simulink model "GPC_GUI"  (R2015b)
settings: Solver=FixedStepAuto  StartTime=0.0  StopTime=100  FixedStep=0.2  RelTol=1e-3
settings Model: Creator=E:\GreenSoftware\TDZ\User\  LastModifiedBy=TroyLab

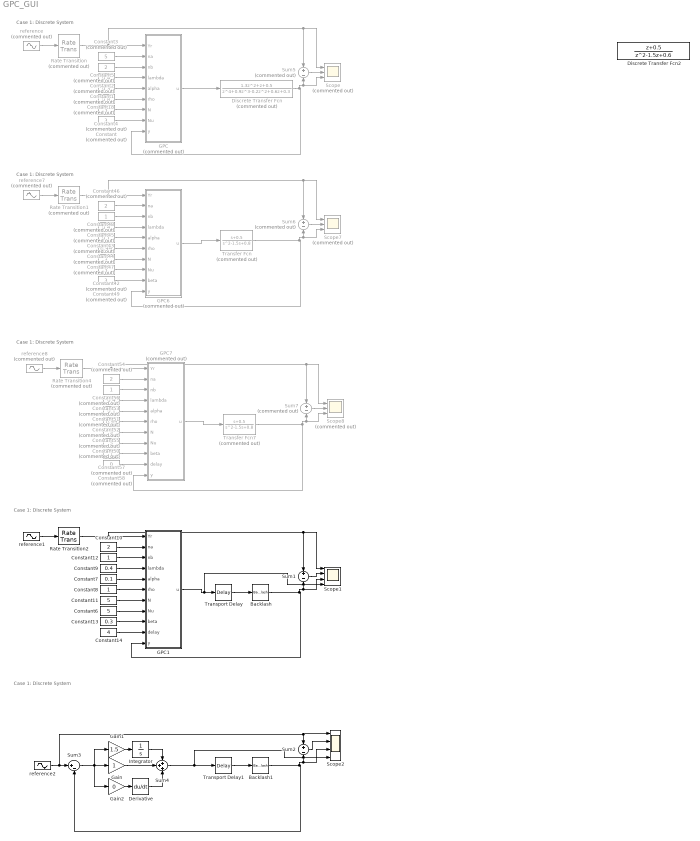
== system GPC_GUI ==
  note: Case 1: Discrete System
  note: Case 1: Discrete System
  note: Case 1: Discrete System
  note: Case 1: Discrete System
  note: Case 1: Discrete System
  Backlash : Backlash  BacklashWidth=1.5
  Backlash1 : Backlash
  Constant{,4,42,47,49} (5 alike) : Constant  Commented=on  Value=3
  Constant1 : Constant  Commented=on  Value=0.3
  Constant10 : Constant  Value=2
  Constant11 : Constant  Value=5
  Constant12 : Constant
  Constant13 : Constant  Value=0.3
  Constant14 : Constant  Value=4
  Constant18 : Constant  Commented=on  Value=0.8
  Constant2 : Constant  Commented=on  Value=0.4
  Constant3 : Constant  Commented=on  Value=5
  Constant43 : Constant  Commented=on  Value=0.1
  Constant44 : Constant  Commented=on  Value=0.99
  Constant45 : Constant  Commented=on  Value=0.4
  Constant46 : Constant  Commented=on  Value=2
  Constant48 : Constant  Commented=on
  Constant5 : Constant  Commented=on  Value=2
  Constant50 : Constant  Commented=on  Value=5
  Constant51 : Constant  Commented=on  Value=0.1
  Constant52 : Constant  Commented=on  Value=0.99
  Constant53 : Constant  Commented=on  Value=0.4
  Constant54 : Constant  Commented=on  Value=2
  Constant55 : Constant  Commented=on  Value=5
  Constant56 : Constant  Commented=on
  Constant57 : Constant  Commented=on
  Constant58 : Constant  Commented=on  Value=0
  Constant6 : Constant  Value=5
  Constant7 : Constant  Value=0.1
  Constant8 : Constant
  Constant9 : Constant  Value=0.4
  Derivative : Derivative
  Discrete Transfer Fcn : DiscreteTransferFcn  Commented=on  Numerator=[1.3, 1, 0.5]  Denominator=[1, 0.9, -0.2, 0.6, 0.3]
  Discrete Transfer Fcn2 : DiscreteTransferFcn  Numerator=[1, 0.5]  Denominator=[1, -1.5, 0.6]
  GPC : MATLAB Function  Commented=on  TreatAsAtomicUnit=on
  GPC1 : MATLAB Function  TreatAsAtomicUnit=on
  GPC6 : MATLAB Function  Commented=on  TreatAsAtomicUnit=on
  GPC7 : MATLAB Function  Commented=on  TreatAsAtomicUnit=on
  Gain : Gain
  Gain1 : Gain  Gain=1.5
  Gain2 : Gain  Gain=0
  Integrator : Integrator
  Rate Transition : RateTransition  Commented=on
  Rate Transition1 : RateTransition  Commented=on
  Rate Transition2 : RateTransition
  Rate Transition4 : RateTransition  Commented=on
  Scope : Scope  Commented=on  NumInputPorts=3
  Scope1 : Scope  NumInputPorts=4
  Scope2 : Scope  NumInputPorts=4
  Scope7 : Scope  Commented=on  NumInputPorts=3
  Scope8 : Scope  Commented=on  NumInputPorts=3
  Sum1 : Sum  Inputs=+|-
  Sum2 : Sum  Inputs=+|-
  Sum3 : Sum  Inputs=|+-
  Sum4 : Sum  Inputs=+++
  Sum5 : Sum  Commented=on  Inputs=+|-
  Sum6 : Sum  Commented=on  Inputs=+|-
  Sum7 : Sum  Commented=on  Inputs=+|-
  Transfer Fcn : TransferFcn  Commented=on  Numerator=[1, 0.5]  Denominator=[1, -1.5, 0.8]
  Transfer Fcn7 : TransferFcn  Commented=on  Numerator=[1, 0.5]  Denominator=[1, -1.5, 0.8]
  Transport Delay : TransportDelay  DelayTime=0.6
  Transport Delay1 : TransportDelay  DelayTime=0.6
  reference : Sin  Commented=on  Frequency=0.2  Phase=pi/4  SampleTime=0
  reference1 : Sin  Amplitude=10  Frequency=0.5  Phase=pi/4  SampleTime=0
  reference2 : Sin  Amplitude=10  Frequency=0.5  Phase=pi/4  SampleTime=0
  reference7 : Sin  Commented=on  Amplitude=10  Frequency=0.5  Phase=pi/4  SampleTime=0
  reference8 : Sin  Commented=on  Amplitude=10  Frequency=0.5  Phase=pi/4  SampleTime=0
  wires:
  reference/1 -> Rate Transition/1
  Constant/1 -> GPC/8(Nu)
  Constant1/1 -> GPC/5(alpha)
  Constant2/1 -> GPC/4(lambda)
  Constant3/1 -> GPC/2(na)
  Constant4/1 -> GPC/7(N)
  Constant5/1 -> GPC/3(nb)
  Discrete Transfer Fcn/1 -> Sum5/2, Scope/3, GPC/9(y)
  Rate Transition/1 -> Sum5/1, Scope/1, GPC/1(Yr)
  GPC/1(u) -> Discrete Transfer Fcn/1
  Transport Delay/1 -> Backlash/1
  Constant18/1 -> GPC/6(rho)
  Sum5/1 -> Scope/2
  reference7/1 -> Rate Transition1/1
  Constant42/1 -> GPC6/8(Nu)
  Constant43/1 -> GPC6/5(alpha)
  Constant45/1 -> GPC6/4(lambda)
  Constant46/1 -> GPC6/2(na)
  Constant47/1 -> GPC6/7(N)
  Constant48/1 -> GPC6/3(nb)
  Transfer Fcn/1 -> GPC6/10(y), Scope7/3, Sum6/2
  Rate Transition1/1 -> GPC6/1(Yr), Scope7/1, Sum6/1
  GPC6/1(u) -> Transfer Fcn/1
  Constant44/1 -> GPC6/6(rho)
  Sum6/1 -> Scope7/2
  Constant49/1 -> GPC6/9(beta)
  reference8/1 -> Rate Transition4/1
  Constant50/1 -> GPC7/8(Nu)
  Constant51/1 -> GPC7/5(alpha)
  Constant53/1 -> GPC7/4(lambda)
  Constant54/1 -> GPC7/2(na)
  Constant55/1 -> GPC7/7(N)
  Constant56/1 -> GPC7/3(nb)
  Transfer Fcn7/1 -> Sum7/2, Scope8/3, GPC7/11(y)
  Rate Transition4/1 -> Sum7/1, Scope8/1, GPC7/1(Yr)
  GPC7/1(u) -> Transfer Fcn7/1
  Constant52/1 -> GPC7/6(rho)
  Sum7/1 -> Scope8/2
  Constant57/1 -> GPC7/9(beta)
  Constant58/1 -> GPC7/10(delay)
  reference1/1 -> Rate Transition2/1
  Constant6/1 -> GPC1/8(Nu)
  Constant7/1 -> GPC1/5(alpha)
  Constant9/1 -> GPC1/4(lambda)
  Constant10/1 -> GPC1/2(na)
  Constant11/1 -> GPC1/7(N)
  Constant12/1 -> GPC1/3(nb)
  Backlash/1 -> GPC1/11(y), Scope1/3, Sum1/2
  Rate Transition2/1 -> GPC1/1(Yr), Scope1/1, Sum1/1
  GPC1/1(u) -> Scope1/4, Transport Delay/1
  Constant8/1 -> GPC1/6(rho)
  Sum1/1 -> Scope1/2
  Constant13/1 -> GPC1/9(beta)
  Constant14/1 -> GPC1/10(delay)
  Transport Delay1/1 -> Backlash1/1
  reference2/1 -> Sum2/1, Scope2/1, Sum3/1
  Backlash1/1 -> Sum3/2, Sum2/2, Scope2/3
  Sum4/1 -> Scope2/4, Transport Delay1/1
  Sum2/1 -> Scope2/2
  Gain2/1 -> Derivative/1
  Gain1/1 -> Integrator/1
  Gain/1 -> Sum4/2
  Integrator/1 -> Sum4/1
  Derivative/1 -> Sum4/3
  Sum3/1 -> Gain1/1, Gain/1, Gain2/1

== matlab function GPC_GUI/GPC1 ==
  data: Yr input; na input; nb input; lambda input; alpha input; rho input; N input; Nu input; beta input; delay input; u output; y input
function u   = fcn(Yr, na, nb, lambda, alpha, rho, N, Nu, beta, delay, y)
    persistent hatU Y hatA hatB theta P;
	na  = int8(na);
	nb  = int8(nb);
    N   = int8(N);
    delay = int8(delay);
    Nu  = int8(Nu);
    if isempty(hatU)
        Y     = zeros(na + 1, 1);
        P     = 100 * eye(na + nb + 1);
        theta = cumprod(0.7*ones(na + nb + 1, 1));
        hatU  = zeros(nb + 2, 1);
    end

	%    |y(k)    |          |u(k-1)     |
	%    |y(y-1)  |          |u(y-2)     |
	% Y =|y(y-2)  |  ,  U =  |u(y-3)     |  ,
	%    |...     |          |...        |
	%    |y(y-na) |          |u(y-nb - 1)|
    % Phi = flipud([diff(hatU); -diff(Y)]);
	% Phi = [diff(Y); -diff(hatU)];
	% Phi = [diff(Y); flipud(diff(hatU))];
	Phi = [diff(Y); -diff(hatU)];
    % Y = [Y(2:na+1); y];
	Y = [y; Y(1:na)];
    % deltaY = Y(end) - Y(end-1);
	deltaY = Y(1) - Y(2);
    theta = theta + (rho + Phi' * P * Phi)\ P * Phi * (deltaY - Phi' * theta);
    P     = (P-(rho+Phi'*P*Phi)\P*Phi*Phi'*P)/rho;

    hatA = [1 theta(1:na)'];		% estimation of coeffeciences of A, row-vector!
    hatB = theta(na+1:end)';		% estimation of coeffeciences of B, row-vector!

    % ------------------------------------
    % Estimate E,F,G,H using diophantine iteration
    % ------------------------------------
    % Solve the Diophantine eqaution 
    % $1      = E_{j}A\Delta+BF_{j}$
    % $E_{j}B = G_{j}+z^{-j}H_{J}$
    [F, H, g] = Diophantine(conv([1, -1],hatA), hatB, N);
    % Y0 = F * Y(end:-1:1)+H * flipud(diff(hatU(2:end)));
    % Y0 = F * Y+H * flipud(diff(hatU(2:end)));
    Y0 = F * Y-H * diff(hatU(1:end-1));

    GG=zeros(N,Nu);
    for n=1:Nu
        GG(n:N,n)=g(1:N-n+1);
    end

    Gain      = (GG'*GG+lambda*eye(Nu))\GG';		% actually, we need only the first line of the Gain matrix, thus 
    Gain      = Gain(1,:);

    % Yd = (Y(size(hatA,2)) - Yr) * cumprod( alpha * ones(N, 1)) + Yr;
    y_cur = 0;
    if delay > 0
        y_cur = Y0(delay);
    else
        y_cur = Y(1);
    end
    Yd = (y_cur - Yr) * cumprod( alpha * ones(N, 1)) + Yr;
    deltaU = beta * Gain * (Yd - Y0);
    % u = hatU(end) + deltaU;
    u = hatU(1) + deltaU;
    % hatU= [hatU(2:nb + 2); u];
    hatU= [u; hatU(1:nb + 1)];
end

function [F, H, g] = Diophantine(A, B, N)
    % Since in Simulink, dynamic expand the matrix is not supported
    % Preallocate space
    e = zeros(1, N);
    g = zeros(1, N);
    F = zeros(N, length(A) - 1);
    H = zeros(N, length(B) - 1);
    % assign values
    e(1)  = 1;
	f  = -A(2:end);
 	g(1)  = e(1)*B(1);
 	h  = B(2:end);
    
	H(1,:) = h;
	F(1,:) = f;

	% Prediction for n steps
	for n=2:N
        ej = f(1);
        % $E_{j+1} = E_j + e_j z^{-j}$
        e(n) = ej;
		% $F_{j+1}=z[F_{j}-e_{j}A]$
		f = [f(2:end), 0]  - A(2:end) * ej;
        g(n) = ej*B(1)+h(1);
		h = [h(2:end), 0] + ej * B(2:end);
        
		F(n,:) = f;
		H(n,:) = h;
	end
end

== matlab function GPC_GUI/GPC ==
  data: Yr input; na input; nb input; lambda input; alpha input; rho input; N input; Nu input; u output; y input
function u  = fcn(Yr, na, nb, lambda, alpha, rho, N, Nu, y)
    persistent hatU Y hatA hatB theta P;
	na  = int8(na);
	nb  = int8(nb);
    N   = int8(N);
    Nu  = int8(Nu);
    if isempty(hatU)
        Y     = zeros(na + 1, 1);
        P     = 100 * eye(na + nb + 1);
        theta = cumprod(0.7*ones(na + nb + 1, 1));
        hatU  = zeros(nb + 2, 1);
    end

    Phi = flipud([diff(hatU); -diff(Y)]);
    Y = [Y(2:na+1); y];
    deltaY = Y(end) - Y(end-1);
    theta = theta + (rho + Phi' * P * Phi)\ P * Phi * (deltaY - Phi' * theta);
    P     = (P-(rho+Phi'*P*Phi)\P*Phi*Phi'*P)/rho;

    hatA = [1 theta(1:na)'];		% estimation of coeffeciences of A, row-vector!
    hatB = theta(na+1:end)';		% estimation of coeffeciences of B, row-vector!

    % ------------------------------------
    % Estimate E,F,G,H using diophantine iteration
    % ------------------------------------
    % Solve the Diophantine eqaution 
    % $1      = E_{j}A\Delta+BF_{j}$
    % $E_{j}B = G_{j}+z^{-j}H_{J}$
    [F, H, g] = Diophantine(conv([1, -1],hatA), hatB, N);
%     Y0 = F * Y(end:-1:1)+H * diff(hatU(2:end));
    Y0 = F * Y(end:-1:1)+H * flipud(diff(hatU(2:end)));

    GG=zeros(N,Nu);
    for n=1:Nu
        GG(n:N,n)=g(1:N-n+1);
    end

    Gain      = (GG'*GG+lambda*eye(Nu))\GG';		% actually, we need only the first line of the Gain matrix, thus 
    Gain      = Gain(1,:);

    Yd = (Y(size(hatA,2)) - Yr) * cumprod( alpha * ones(N, 1)) + Yr;
    deltaU = Gain * (Yd - Y0);
    u = hatU(end) + deltaU;
    hatU= [hatU(2:nb + 2); u];
end

function [F, H, g] = Diophantine(A, B, N)
    % Since in Simulink, dynamic expand the matrix is not supported
    % Preallocate space
    e = zeros(1, N);
    g = zeros(1, N);
    F = zeros(N, length(A) - 1);
    H = zeros(N, length(B) - 1);
    % assign values
    e(1)  = 1;
	f  = -A(2:end);
 	g(1)  = e(1)*B(1);
 	h  = B(2:end);
    
	H(1,:) = h;
	F(1,:) = f;

	% Prediction for n steps
	for n=2:N
        ej = f(1);
        % $E_{j+1} = E_j + e_j z^{-j}$
        e(n) = ej;
		% $F_{j+1}=z[F_{j}-e_{j}A]$
		f = [f(2:end), 0]  - A(2:end) * ej;
        g(n) = ej*B(1)+h(1);
		h = [h(2:end), 0] + ej * B(2:end);
        
		F(n,:) = f;
		H(n,:) = h;
	end
end

== matlab function GPC_GUI/GPC6 ==
  data: Yr input; na input; nb input; lambda input; alpha input; rho input; N input; Nu input; beta input; u output; y input
function u   = fcn(Yr, na, nb, lambda, alpha, rho, N, Nu, beta, y)
    persistent hatU Y hatA hatB theta P;
	na  = int8(na);
	nb  = int8(nb);
    N   = int8(N);
    Nu  = int8(Nu);
    if isempty(hatU)
        Y     = zeros(na + 1, 1);
        P     = 100 * eye(na + nb + 1);
        theta = cumprod(0.7*ones(na + nb + 1, 1));
        hatU  = zeros(nb + 2, 1);
    end

	%    |y(k)    |          |u(k-1)     |
	%    |y(y-1)  |          |u(y-2)     |
	% Y =|y(y-2)  |  ,  U =  |u(y-3)     |  ,
	%    |...     |          |...        |
	%    |y(y-na) |          |u(y-nb - 1)|
    % Phi = flipud([diff(hatU); -diff(Y)]);
	% Phi = [diff(Y); -diff(hatU)];
	% Phi = [diff(Y); flipud(diff(hatU))];
	Phi = [diff(Y); -diff(hatU)];
    % Y = [Y(2:na+1); y];
	Y = [y; Y(1:na)];
    % deltaY = Y(end) - Y(end-1);
	deltaY = Y(1) - Y(2);
    theta = theta + (rho + Phi' * P * Phi)\ P * Phi * (deltaY - Phi' * theta);
    P     = (P-(rho+Phi'*P*Phi)\P*Phi*Phi'*P)/rho;

    hatA = [1 theta(1:na)'];		% estimation of coeffeciences of A, row-vector!
    hatB = theta(na+1:end)';		% estimation of coeffeciences of B, row-vector!

    % ------------------------------------
    % Estimate E,F,G,H using diophantine iteration
    % ------------------------------------
    % Solve the Diophantine eqaution 
    % $1      = E_{j}A\Delta+BF_{j}$
    % $E_{j}B = G_{j}+z^{-j}H_{J}$
    [F, H, g] = Diophantine(conv([1, -1],hatA), hatB, N);
    % Y0 = F * Y(end:-1:1)+H * flipud(diff(hatU(2:end)));
    % Y0 = F * Y+H * flipud(diff(hatU(2:end)));
    Y0 = F * Y-H * diff(hatU(1:end-1));

    GG=zeros(N,Nu);
    for n=1:Nu
        GG(n:N,n)=g(1:N-n+1);
    end

    Gain      = (GG'*GG+lambda*eye(Nu))\GG';		% actually, we need only the first line of the Gain matrix, thus 
    Gain      = Gain(1,:);

    % Yd = (Y(size(hatA,2)) - Yr) * cumprod( alpha * ones(N, 1)) + Yr;
    Yd = (Y(1) - Yr) * cumprod( alpha * ones(N, 1)) + Yr;
    deltaU = beta * Gain * (Yd - Y0);
    % u = hatU(end) + deltaU;
    u = hatU(1) + deltaU;
    % hatU= [hatU(2:nb + 2); u];
    hatU= [u; hatU(1:nb + 1)];
end

function [F, H, g] = Diophantine(A, B, N)
    % Since in Simulink, dynamic expand the matrix is not supported
    % Preallocate space
    e = zeros(1, N);
    g = zeros(1, N);
    F = zeros(N, length(A) - 1);
    H = zeros(N, length(B) - 1);
    % assign values
    e(1)  = 1;
	f  = -A(2:end);
 	g(1)  = e(1)*B(1);
 	h  = B(2:end);
    
	H(1,:) = h;
	F(1,:) = f;

	% Prediction for n steps
	for n=2:N
        ej = f(1);
        % $E_{j+1} = E_j + e_j z^{-j}$
        e(n) = ej;
		% $F_{j+1}=z[F_{j}-e_{j}A]$
		f = [f(2:end), 0]  - A(2:end) * ej;
        g(n) = ej*B(1)+h(1);
		h = [h(2:end), 0] + ej * B(2:end);
        
		F(n,:) = f;
		H(n,:) = h;
	end
end

== matlab function GPC_GUI/GPC7 ==
  data: Yr input; na input; nb input; lambda input; alpha input; rho input; N input; Nu input; beta input; delay input; u output; y input
function u   = fcn(Yr, na, nb, lambda, alpha, rho, N, Nu, beta, delay, y)
    persistent hatU Y hatA hatB theta P;
	na  = int8(na);
	nb  = int8(nb);
    N   = int8(N);
    delay = int8(delay);
    Nu  = int8(Nu);
    if isempty(hatU)
        Y     = zeros(na + 1, 1);
        P     = 100 * eye(na + nb + 1);
        theta = cumprod(0.7*ones(na + nb + 1, 1));
        hatU  = zeros(nb + 2, 1);
    end

	%    |y(k)    |          |u(k-1)     |
	%    |y(y-1)  |          |u(y-2)     |
	% Y =|y(y-2)  |  ,  U =  |u(y-3)     |  ,
	%    |...     |          |...        |
	%    |y(y-na) |          |u(y-nb - 1)|
    % Phi = flipud([diff(hatU); -diff(Y)]);
	% Phi = [diff(Y); -diff(hatU)];
	% Phi = [diff(Y); flipud(diff(hatU))];
	Phi = [diff(Y); -diff(hatU)];
    % Y = [Y(2:na+1); y];
	Y = [y; Y(1:na)];
    % deltaY = Y(end) - Y(end-1);
	deltaY = Y(1) - Y(2);
    theta = theta + (rho + Phi' * P * Phi)\ P * Phi * (deltaY - Phi' * theta);
    P     = (P-(rho+Phi'*P*Phi)\P*Phi*Phi'*P)/rho;

    hatA = [1 theta(1:na)'];		% estimation of coeffeciences of A, row-vector!
    hatB = theta(na+1:end)';		% estimation of coeffeciences of B, row-vector!

    % ------------------------------------
    % Estimate E,F,G,H using diophantine iteration
    % ------------------------------------
    % Solve the Diophantine eqaution 
    % $1      = E_{j}A\Delta+BF_{j}$
    % $E_{j}B = G_{j}+z^{-j}H_{J}$
    [F, H, g] = Diophantine(conv([1, -1],hatA), hatB, N);
    % Y0 = F * Y(end:-1:1)+H * flipud(diff(hatU(2:end)));
    % Y0 = F * Y+H * flipud(diff(hatU(2:end)));
    Y0 = F * Y-H * diff(hatU(1:end-1));

    GG=zeros(N,Nu);
    for n=1:Nu
        GG(n:N,n)=g(1:N-n+1);
    end

    Gain      = (GG'*GG+lambda*eye(Nu))\GG';		% actually, we need only the first line of the Gain matrix, thus 
    Gain      = Gain(1,:);

    % Yd = (Y(size(hatA,2)) - Yr) * cumprod( alpha * ones(N, 1)) + Yr;
    y_cur = 0;
    if delay > 0
        y_cur = Y0(delay);
    else
        y_cur = Y(1);
    end
    Yd = (y_cur - Yr) * cumprod( alpha * ones(N, 1)) + Yr;
    deltaU = beta * Gain * (Yd - Y0);
    % u = hatU(end) + deltaU;
    u = hatU(1) + deltaU;
    % hatU= [hatU(2:nb + 2); u];
    hatU= [u; hatU(1:nb + 1)];
end

function [F, H, g] = Diophantine(A, B, N)
    % Since in Simulink, dynamic expand the matrix is not supported
    % Preallocate space
    e = zeros(1, N);
    g = zeros(1, N);
    F = zeros(N, length(A) - 1);
    H = zeros(N, length(B) - 1);
    % assign values
    e(1)  = 1;
	f  = -A(2:end);
 	g(1)  = e(1)*B(1);
 	h  = B(2:end);
    
	H(1,:) = h;
	F(1,:) = f;

	% Prediction for n steps
	for n=2:N
        ej = f(1);
        % $E_{j+1} = E_j + e_j z^{-j}$
        e(n) = ej;
		% $F_{j+1}=z[F_{j}-e_{j}A]$
		f = [f(2:end), 0]  - A(2:end) * ej;
        g(n) = ej*B(1)+h(1);
		h = [h(2:end), 0] + ej * B(2:end);
        
		F(n,:) = f;
		H(n,:) = h;
	end
end
